simulink model "orion_casestudy_4"  (R2023a)
settings: Solver=VariableStepAuto  StartTime=0.0  StopTime=30  RelTol=1e-3
InitFcn:
  | RandStream.setGlobalStream(RandStream('mt19937ar','seed',sum(100*clock)));
undefined symbols (not defined in the file or in its folder): m, n
(part 1 of 2)
settings Model: Creator=simon  LastModifiedBy=simon
settings OptimizationCC: AccelVerboseBuild=on
settings DebuggingCC: UnderSpecifiedDataTypeMsg=warning  UnderSpecifiedDimensionMsg=warning

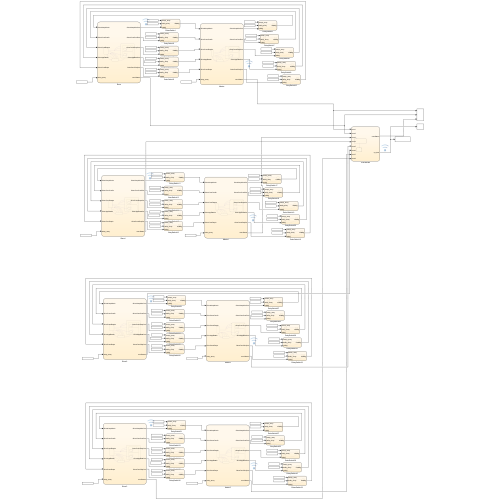
[thumbnail: Simulink's stored preview of the top-level diagram]
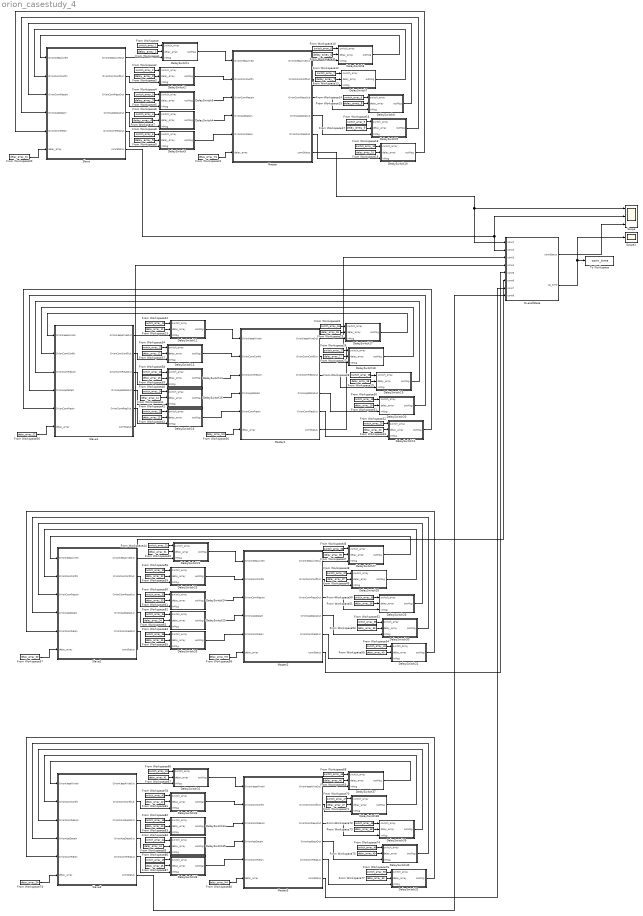
== system orion_casestudy_4 ==
  DelaySwitch1 : Stateflow chart  TreatAsAtomicUnit=on
  DelaySwitch10 : Stateflow chart  TreatAsAtomicUnit=on
  DelaySwitch11 : Stateflow chart  TreatAsAtomicUnit=on
  DelaySwitch12 : Stateflow chart  TreatAsAtomicUnit=on
  DelaySwitch13 : Stateflow chart  TreatAsAtomicUnit=on
  DelaySwitch14 : Stateflow chart  TreatAsAtomicUnit=on
  DelaySwitch15 : Stateflow chart  TreatAsAtomicUnit=on
  DelaySwitch16 : Stateflow chart  TreatAsAtomicUnit=on
  DelaySwitch17 : Stateflow chart  TreatAsAtomicUnit=on
  DelaySwitch18 : Stateflow chart  TreatAsAtomicUnit=on
  DelaySwitch19 : Stateflow chart  TreatAsAtomicUnit=on
  DelaySwitch2 : Stateflow chart  TreatAsAtomicUnit=on
  DelaySwitch20 : Stateflow chart  TreatAsAtomicUnit=on
  DelaySwitch21 : Stateflow chart  TreatAsAtomicUnit=on
  DelaySwitch22 : Stateflow chart  TreatAsAtomicUnit=on
  DelaySwitch23 : Stateflow chart  TreatAsAtomicUnit=on
  DelaySwitch24 : Stateflow chart  TreatAsAtomicUnit=on
  DelaySwitch25 : Stateflow chart  TreatAsAtomicUnit=on
  DelaySwitch26 : Stateflow chart  TreatAsAtomicUnit=on
  DelaySwitch27 : Stateflow chart  TreatAsAtomicUnit=on
  DelaySwitch28 : Stateflow chart  TreatAsAtomicUnit=on
  DelaySwitch29 : Stateflow chart  TreatAsAtomicUnit=on
  DelaySwitch3 : Stateflow chart  TreatAsAtomicUnit=on
  DelaySwitch30 : Stateflow chart  TreatAsAtomicUnit=on
  DelaySwitch31 : Stateflow chart  TreatAsAtomicUnit=on
  DelaySwitch32 : Stateflow chart  TreatAsAtomicUnit=on
  DelaySwitch33 : Stateflow chart  TreatAsAtomicUnit=on
  DelaySwitch34 : Stateflow chart  TreatAsAtomicUnit=on
  DelaySwitch35 : Stateflow chart  TreatAsAtomicUnit=on
  DelaySwitch36 : Stateflow chart  TreatAsAtomicUnit=on
  DelaySwitch37 : Stateflow chart  TreatAsAtomicUnit=on
  DelaySwitch38 : Stateflow chart  TreatAsAtomicUnit=on
  DelaySwitch39 : Stateflow chart  TreatAsAtomicUnit=on
  DelaySwitch4 : Stateflow chart  TreatAsAtomicUnit=on
  DelaySwitch40 : Stateflow chart  TreatAsAtomicUnit=on
  DelaySwitch5 : Stateflow chart  TreatAsAtomicUnit=on
  DelaySwitch6 : Stateflow chart  TreatAsAtomicUnit=on
  DelaySwitch7 : Stateflow chart  TreatAsAtomicUnit=on
  DelaySwitch8 : Stateflow chart  TreatAsAtomicUnit=on
  DelaySwitch9 : Stateflow chart  TreatAsAtomicUnit=on
  From Workspace : FromWorkspace  VariableName=switch_array_1  SampleTime=-1  Interpolate=off  ZeroCross=off  OutputAfterFinalValue=Holding final value
  From Workspace1 : FromWorkspace  VariableName=delay_array_1  SampleTime=-1  Interpolate=off  ZeroCross=off  OutputAfterFinalValue=Holding final value
  From Workspace10 : FromWorkspace  VariableName=switch_array_6  SampleTime=-1  Interpolate=off  ZeroCross=off  OutputAfterFinalValue=Holding final value
  From Workspace11 : FromWorkspace  VariableName=delay_array_6  SampleTime=-1  Interpolate=off  ZeroCross=off  OutputAfterFinalValue=Holding final value
  From Workspace12 : FromWorkspace  VariableName=switch_array_7  SampleTime=-1  Interpolate=off  ZeroCross=off  OutputAfterFinalValue=Holding final value
  From Workspace13 : FromWorkspace  VariableName=delay_array_7  SampleTime=-1  Interpolate=off  ZeroCross=off  OutputAfterFinalValue=Holding final value
  From Workspace14 : FromWorkspace  VariableName=switch_array_8  SampleTime=-1  Interpolate=off  ZeroCross=off  OutputAfterFinalValue=Holding final value
  From Workspace15 : FromWorkspace  VariableName=delay_array_8  SampleTime=-1  Interpolate=off  ZeroCross=off  OutputAfterFinalValue=Holding final value
  From Workspace16 : FromWorkspace  VariableName=switch_array_9  SampleTime=-1  Interpolate=off  ZeroCross=off  OutputAfterFinalValue=Holding final value
  From Workspace17 : FromWorkspace  VariableName=delay_array_9  SampleTime=-1  Interpolate=off  ZeroCross=off  OutputAfterFinalValue=Holding final value
  From Workspace18 : FromWorkspace  VariableName=switch_array_10  SampleTime=-1  Interpolate=off  ZeroCross=off  OutputAfterFinalValue=Holding final value
  From Workspace19 : FromWorkspace  VariableName=delay_array_10  SampleTime=-1  Interpolate=off  ZeroCross=off  OutputAfterFinalValue=Holding final value
  From Workspace2 : FromWorkspace  VariableName=switch_array_2  SampleTime=-1  Interpolate=off  ZeroCross=off  OutputAfterFinalValue=Holding final value
  From Workspace20 : FromWorkspace  VariableName=delay_array_S1  SampleTime=-1  Interpolate=off  ZeroCross=off  OutputAfterFinalValue=Holding final value
  From Workspace21 : FromWorkspace  VariableName=delay_array_M1  SampleTime=-1  Interpolate=off  ZeroCross=off  OutputAfterFinalValue=Holding final value
  From Workspace22 : FromWorkspace  VariableName=switch_array_11  SampleTime=-1  Interpolate=off  ZeroCross=off  OutputAfterFinalValue=Holding final value
  From Workspace23 : FromWorkspace  VariableName=delay_array_11  SampleTime=-1  Interpolate=off  ZeroCross=off  OutputAfterFinalValue=Holding final value
  From Workspace24 : FromWorkspace  VariableName=switch_array_16  SampleTime=-1  Interpolate=off  ZeroCross=off  OutputAfterFinalValue=Holding final value
  From Workspace25 : FromWorkspace  VariableName=delay_array_16  SampleTime=-1  Interpolate=off  ZeroCross=off  OutputAfterFinalValue=Holding final value
  From Workspace26 : FromWorkspace  VariableName=switch_array_17  SampleTime=-1  Interpolate=off  ZeroCross=off  OutputAfterFinalValue=Holding final value
  From Workspace27 : FromWorkspace  VariableName=delay_array_17  SampleTime=-1  Interpolate=off  ZeroCross=off  OutputAfterFinalValue=Holding final value
  From Workspace28 : FromWorkspace  VariableName=switch_array_18  SampleTime=-1  Interpolate=off  ZeroCross=off  OutputAfterFinalValue=Holding final value
  From Workspace29 : FromWorkspace  VariableName=delay_array_18  SampleTime=-1  Interpolate=off  ZeroCross=off  OutputAfterFinalValue=Holding final value
  From Workspace3 : FromWorkspace  VariableName=delay_array_2  SampleTime=-1  Interpolate=off  ZeroCross=off  OutputAfterFinalValue=Holding final value
  From Workspace30 : FromWorkspace  VariableName=switch_array_19  SampleTime=-1  Interpolate=off  ZeroCross=off  OutputAfterFinalValue=Holding final value
  From Workspace31 : FromWorkspace  VariableName=delay_array_19  SampleTime=-1  Interpolate=off  ZeroCross=off  OutputAfterFinalValue=Holding final value
  From Workspace32 : FromWorkspace  VariableName=switch_array_20  SampleTime=-1  Interpolate=off  ZeroCross=off  OutputAfterFinalValue=Holding final value
  From Workspace33 : FromWorkspace  VariableName=delay_array_20  SampleTime=-1  Interpolate=off  ZeroCross=off  OutputAfterFinalValue=Holding final value
  From Workspace34 : FromWorkspace  VariableName=switch_array_12  SampleTime=-1  Interpolate=off  ZeroCross=off  OutputAfterFinalValue=Holding final value
  From Workspace35 : FromWorkspace  VariableName=delay_array_S2  SampleTime=-1  Interpolate=off  ZeroCross=off  OutputAfterFinalValue=Holding final value
  From Workspace36 : FromWorkspace  VariableName=delay_array_M2  SampleTime=-1  Interpolate=off  ZeroCross=off  OutputAfterFinalValue=Holding final value
  From Workspace37 : FromWorkspace  VariableName=delay_array_12  SampleTime=-1  Interpolate=off  ZeroCross=off  OutputAfterFinalValue=Holding final value
  From Workspace38 : FromWorkspace  VariableName=switch_array_13  SampleTime=-1  Interpolate=off  ZeroCross=off  OutputAfterFinalValue=Holding final value
  From Workspace39 : FromWorkspace  VariableName=delay_array_13  SampleTime=-1  Interpolate=off  ZeroCross=off  OutputAfterFinalValue=Holding final value
  From Workspace4 : FromWorkspace  VariableName=switch_array_3  SampleTime=-1  Interpolate=off  ZeroCross=off  OutputAfterFinalValue=Holding final value
  From Workspace40 : FromWorkspace  VariableName=switch_array_14  SampleTime=-1  Interpolate=off  ZeroCross=off  OutputAfterFinalValue=Holding final value
  From Workspace41 : FromWorkspace  VariableName=delay_array_14  SampleTime=-1  Interpolate=off  ZeroCross=off  OutputAfterFinalValue=Holding final value
  From Workspace42 : FromWorkspace  VariableName=switch_array_15  SampleTime=-1  Interpolate=off  ZeroCross=off  OutputAfterFinalValue=Holding final value
  From Workspace43 : FromWorkspace  VariableName=delay_array_15  SampleTime=-1  Interpolate=off  ZeroCross=off  OutputAfterFinalValue=Holding final value
  From Workspace44 : FromWorkspace  VariableName=switch_array_31  SampleTime=-1  Interpolate=off  ZeroCross=off  OutputAfterFinalValue=Holding final value
  From Workspace45 : FromWorkspace  VariableName=delay_array_31  SampleTime=-1  Interpolate=off  ZeroCross=off  OutputAfterFinalValue=Holding final value
  From Workspace46 : FromWorkspace  VariableName=switch_array_36  SampleTime=-1  Interpolate=off  ZeroCross=off  OutputAfterFinalValue=Holding final value
  From Workspace47 : FromWorkspace  VariableName=delay_array_36  SampleTime=-1  Interpolate=off  ZeroCross=off  OutputAfterFinalValue=Holding final value
  From Workspace48 : FromWorkspace  VariableName=switch_array_37  SampleTime=-1  Interpolate=off  ZeroCross=off  OutputAfterFinalValue=Holding final value
  From Workspace49 : FromWorkspace  VariableName=delay_array_37  SampleTime=-1  Interpolate=off  ZeroCross=off  OutputAfterFinalValue=Holding final value
  From Workspace5 : FromWorkspace  VariableName=delay_array_3  SampleTime=-1  Interpolate=off  ZeroCross=off  OutputAfterFinalValue=Holding final value
  From Workspace50 : FromWorkspace  VariableName=switch_array_38  SampleTime=-1  Interpolate=off  ZeroCross=off  OutputAfterFinalValue=Holding final value
  From Workspace51 : FromWorkspace  VariableName=delay_array_38  SampleTime=-1  Interpolate=off  ZeroCross=off  OutputAfterFinalValue=Holding final value
  From Workspace52 : FromWorkspace  VariableName=switch_array_39  SampleTime=-1  Interpolate=off  ZeroCross=off  OutputAfterFinalValue=Holding final value
  From Workspace53 : FromWorkspace  VariableName=delay_array_39  SampleTime=-1  Interpolate=off  ZeroCross=off  OutputAfterFinalValue=Holding final value
  From Workspace54 : FromWorkspace  VariableName=switch_array_40  SampleTime=-1  Interpolate=off  ZeroCross=off  OutputAfterFinalValue=Holding final value
  From Workspace55 : FromWorkspace  VariableName=delay_array_40  SampleTime=-1  Interpolate=off  ZeroCross=off  OutputAfterFinalValue=Holding final value
  From Workspace56 : FromWorkspace  VariableName=switch_array_32  SampleTime=-1  Interpolate=off  ZeroCross=off  OutputAfterFinalValue=Holding final value
  From Workspace57 : FromWorkspace  VariableName=delay_array_S3  SampleTime=-1  Interpolate=off  ZeroCross=off  OutputAfterFinalValue=Holding final value
  From Workspace58 : FromWorkspace  VariableName=delay_array_M3  SampleTime=-1  Interpolate=off  ZeroCross=off  OutputAfterFinalValue=Holding final value
  From Workspace59 : FromWorkspace  VariableName=delay_array_32  SampleTime=-1  Interpolate=off  ZeroCross=off  OutputAfterFinalValue=Holding final value
  From Workspace6 : FromWorkspace  VariableName=switch_array_4  SampleTime=-1  Interpolate=off  ZeroCross=off  OutputAfterFinalValue=Holding final value
  From Workspace60 : FromWorkspace  VariableName=switch_array_33  SampleTime=-1  Interpolate=off  ZeroCross=off  OutputAfterFinalValue=Holding final value
  From Workspace61 : FromWorkspace  VariableName=delay_array_33  SampleTime=-1  Interpolate=off  ZeroCross=off  OutputAfterFinalValue=Holding final value
  From Workspace62 : FromWorkspace  VariableName=switch_array_34  SampleTime=-1  Interpolate=off  ZeroCross=off  OutputAfterFinalValue=Holding final value
  From Workspace63 : FromWorkspace  VariableName=delay_array_34  SampleTime=-1  Interpolate=off  ZeroCross=off  OutputAfterFinalValue=Holding final value
  From Workspace64 : FromWorkspace  VariableName=switch_array_35  SampleTime=-1  Interpolate=off  ZeroCross=off  OutputAfterFinalValue=Holding final value
  From Workspace65 : FromWorkspace  VariableName=delay_array_35  SampleTime=-1  Interpolate=off  ZeroCross=off  OutputAfterFinalValue=Holding final value
  From Workspace66 : FromWorkspace  VariableName=switch_array_41  SampleTime=-1  Interpolate=off  ZeroCross=off  OutputAfterFinalValue=Holding final value
  From Workspace67 : FromWorkspace  VariableName=delay_array_41  SampleTime=-1  Interpolate=off  ZeroCross=off  OutputAfterFinalValue=Holding final value
  From Workspace68 : FromWorkspace  VariableName=switch_array_46  SampleTime=-1  Interpolate=off  ZeroCross=off  OutputAfterFinalValue=Holding final value
  From Workspace69 : FromWorkspace  VariableName=delay_array_46  SampleTime=-1  Interpolate=off  ZeroCross=off  OutputAfterFinalValue=Holding final value
  From Workspace7 : FromWorkspace  VariableName=delay_array_4  SampleTime=-1  Interpolate=off  ZeroCross=off  OutputAfterFinalValue=Holding final value
  From Workspace70 : FromWorkspace  VariableName=switch_array_47  SampleTime=-1  Interpolate=off  ZeroCross=off  OutputAfterFinalValue=Holding final value
  From Workspace71 : FromWorkspace  VariableName=delay_array_47  SampleTime=-1  Interpolate=off  ZeroCross=off  OutputAfterFinalValue=Holding final value
  From Workspace72 : FromWorkspace  VariableName=switch_array_48  SampleTime=-1  Interpolate=off  ZeroCross=off  OutputAfterFinalValue=Holding final value
  From Workspace73 : FromWorkspace  VariableName=delay_array_48  SampleTime=-1  Interpolate=off  ZeroCross=off  OutputAfterFinalValue=Holding final value
  From Workspace74 : FromWorkspace  VariableName=switch_array_49  SampleTime=-1  Interpolate=off  ZeroCross=off  OutputAfterFinalValue=Holding final value
  From Workspace75 : FromWorkspace  VariableName=delay_array_49  SampleTime=-1  Interpolate=off  ZeroCross=off  OutputAfterFinalValue=Holding final value
  From Workspace76 : FromWorkspace  VariableName=switch_array_50  SampleTime=-1  Interpolate=off  ZeroCross=off  OutputAfterFinalValue=Holding final value
  From Workspace77 : FromWorkspace  VariableName=delay_array_50  SampleTime=-1  Interpolate=off  ZeroCross=off  OutputAfterFinalValue=Holding final value
  From Workspace78 : FromWorkspace  VariableName=switch_array_42  SampleTime=-1  Interpolate=off  ZeroCross=off  OutputAfterFinalValue=Holding final value
  From Workspace79 : FromWorkspace  VariableName=delay_array_S4  SampleTime=-1  Interpolate=off  ZeroCross=off  OutputAfterFinalValue=Holding final value
  From Workspace8 : FromWorkspace  VariableName=switch_array_5  SampleTime=-1  Interpolate=off  ZeroCross=off  OutputAfterFinalValue=Holding final value
  From Workspace80 : FromWorkspace  VariableName=delay_array_M4  SampleTime=-1  Interpolate=off  ZeroCross=off  OutputAfterFinalValue=Holding final value
  From Workspace81 : FromWorkspace  VariableName=delay_array_42  SampleTime=-1  Interpolate=off  ZeroCross=off  OutputAfterFinalValue=Holding final value
  From Workspace82 : FromWorkspace  VariableName=switch_array_43  SampleTime=-1  Interpolate=off  ZeroCross=off  OutputAfterFinalValue=Holding final value
  From Workspace83 : FromWorkspace  VariableName=delay_array_43  SampleTime=-1  Interpolate=off  ZeroCross=off  OutputAfterFinalValue=Holding final value
  From Workspace84 : FromWorkspace  VariableName=switch_array_44  SampleTime=-1  Interpolate=off  ZeroCross=off  OutputAfterFinalValue=Holding final value
  From Workspace85 : FromWorkspace  VariableName=delay_array_44  SampleTime=-1  Interpolate=off  ZeroCross=off  OutputAfterFinalValue=Holding final value
  From Workspace86 : FromWorkspace  VariableName=switch_array_45  SampleTime=-1  Interpolate=off  ZeroCross=off  OutputAfterFinalValue=Holding final value
  From Workspace87 : FromWorkspace  VariableName=delay_array_45  SampleTime=-1  Interpolate=off  ZeroCross=off  OutputAfterFinalValue=Holding final value
  From Workspace9 : FromWorkspace  VariableName=delay_array_5  SampleTime=-1  Interpolate=off  ZeroCross=off  OutputAfterFinalValue=Holding final value
  Master : Stateflow chart  TreatAsAtomicUnit=on
      settings: PortSchema="{\"entries\":[{\"content\":{\"sides\":[{\"content\":{\"connectorIds\":[\"In2\",\"In3\",\"In5\",\"In4\",\"In6\",\"In1\"]},\"type\":\"ConnectorPlacement.EquallySpacedRectSide\",\"uuid\":\"93190a42-59cb-4d31-aa72-080cef5549db\"},{\"content\":{\"connectorIds\":[\"Out1\",\"Out2\",\"Out3\",\"Out4\",\"Out5\",\"Out6\"],\"side\":\"RIGHT\"},\"type\":\"ConnectorPlacement.EquallySpacedRectSide\",\"uuid\":\"4a04e977-42e8-4d3e-8e66-86884aeb71d4\"},{\"content\":{\"side\":\"TOP\"},\"type\":\"ConnectorPlacement.EquallySpacedRectSide\",\"uuid\":\"cb7bc3bf-3799-42a3-9f12-c8b4e7be85f7\"},{\"content\":{\"side\":\"BOTTOM\"},\"type\":\"ConnectorPlacement.EquallySpacedRectSide\",\"uuid\":\"934a78a5-af7b-46d0-ad43-c65a76addb63\"}]},\"type\":\"ConnectorPlacement.EquallySpacedConnector\",\"uuid\":\"bab253c4-7746-42e8-9b4d-6fa7ff1cc3b1\"}],\"packageUris\":[\"http://schema.mathworks.com/mf0/Connector/R2020b\"],\"version\":\"1.0\"}"
  Master1 : Stateflow chart  TreatAsAtomicUnit=on
      settings: PortSchema="{\"entries\":[{\"content\":{\"sides\":[{\"content\":{\"connectorIds\":[\"In2\",\"In3\",\"In5\",\"In4\",\"In6\",\"In1\"]},\"type\":\"ConnectorPlacement.EquallySpacedRectSide\",\"uuid\":\"93190a42-59cb-4d31-aa72-080cef5549db\"},{\"content\":{\"connectorIds\":[\"Out1\",\"Out2\",\"Out3\",\"Out4\",\"Out5\",\"Out6\"],\"side\":\"RIGHT\"},\"type\":\"ConnectorPlacement.EquallySpacedRectSide\",\"uuid\":\"4a04e977-42e8-4d3e-8e66-86884aeb71d4\"},{\"content\":{\"side\":\"TOP\"},\"type\":\"ConnectorPlacement.EquallySpacedRectSide\",\"uuid\":\"cb7bc3bf-3799-42a3-9f12-c8b4e7be85f7\"},{\"content\":{\"side\":\"BOTTOM\"},\"type\":\"ConnectorPlacement.EquallySpacedRectSide\",\"uuid\":\"934a78a5-af7b-46d0-ad43-c65a76addb63\"}]},\"type\":\"ConnectorPlacement.EquallySpacedConnector\",\"uuid\":\"bab253c4-7746-42e8-9b4d-6fa7ff1cc3b1\"}],\"packageUris\":[\"http://schema.mathworks.com/mf0/Connector/R2020b\"],\"version\":\"1.0\"}"
  Master2 : Stateflow chart  TreatAsAtomicUnit=on
      settings: PortSchema="{\"entries\":[{\"content\":{\"sides\":[{\"content\":{\"connectorIds\":[\"In2\",\"In3\",\"In5\",\"In4\",\"In6\",\"In1\"]},\"type\":\"ConnectorPlacement.EquallySpacedRectSide\",\"uuid\":\"93190a42-59cb-4d31-aa72-080cef5549db\"},{\"content\":{\"connectorIds\":[\"Out1\",\"Out2\",\"Out3\",\"Out4\",\"Out5\",\"Out6\"],\"side\":\"RIGHT\"},\"type\":\"ConnectorPlacement.EquallySpacedRectSide\",\"uuid\":\"4a04e977-42e8-4d3e-8e66-86884aeb71d4\"},{\"content\":{\"side\":\"TOP\"},\"type\":\"ConnectorPlacement.EquallySpacedRectSide\",\"uuid\":\"cb7bc3bf-3799-42a3-9f12-c8b4e7be85f7\"},{\"content\":{\"side\":\"BOTTOM\"},\"type\":\"ConnectorPlacement.EquallySpacedRectSide\",\"uuid\":\"934a78a5-af7b-46d0-ad43-c65a76addb63\"}]},\"type\":\"ConnectorPlacement.EquallySpacedConnector\",\"uuid\":\"bab253c4-7746-42e8-9b4d-6fa7ff1cc3b1\"}],\"packageUris\":[\"http://schema.mathworks.com/mf0/Connector/R2020b\"],\"version\":\"1.0\"}"
  Master3 : Stateflow chart  TreatAsAtomicUnit=on
      settings: PortSchema="{\"entries\":[{\"content\":{\"sides\":[{\"content\":{\"connectorIds\":[\"In2\",\"In3\",\"In5\",\"In4\",\"In6\",\"In1\"]},\"type\":\"ConnectorPlacement.EquallySpacedRectSide\",\"uuid\":\"93190a42-59cb-4d31-aa72-080cef5549db\"},{\"content\":{\"connectorIds\":[\"Out1\",\"Out2\",\"Out3\",\"Out4\",\"Out5\",\"Out6\"],\"side\":\"RIGHT\"},\"type\":\"ConnectorPlacement.EquallySpacedRectSide\",\"uuid\":\"4a04e977-42e8-4d3e-8e66-86884aeb71d4\"},{\"content\":{\"side\":\"TOP\"},\"type\":\"ConnectorPlacement.EquallySpacedRectSide\",\"uuid\":\"cb7bc3bf-3799-42a3-9f12-c8b4e7be85f7\"},{\"content\":{\"side\":\"BOTTOM\"},\"type\":\"ConnectorPlacement.EquallySpacedRectSide\",\"uuid\":\"934a78a5-af7b-46d0-ad43-c65a76addb63\"}]},\"type\":\"ConnectorPlacement.EquallySpacedConnector\",\"uuid\":\"bab253c4-7746-42e8-9b4d-6fa7ff1cc3b1\"}],\"packageUris\":[\"http://schema.mathworks.com/mf0/Connector/R2020b\"],\"version\":\"1.0\"}"
  OverallState : Stateflow chart  TreatAsAtomicUnit=on
  Scope : Scope  NumInputPorts=3
  Scope1 : Scope
  Slave : Stateflow chart  TreatAsAtomicUnit=on
      settings: PortSchema="{\"entries\":[{\"content\":{\"sides\":[{\"content\":{\"connectorIds\":[\"In1\",\"In5\",\"In3\",\"In2\",\"In4\",\"In6\"]},\"type\":\"ConnectorPlacement.EquallySpacedRectSide\",\"uuid\":\"93190a42-59cb-4d31-aa72-080cef5549db\"},{\"content\":{\"connectorIds\":[\"Out3\",\"Out1\",\"Out2\",\"Out4\",\"Out5\",\"Out6\"],\"side\":\"RIGHT\"},\"type\":\"ConnectorPlacement.EquallySpacedRectSide\",\"uuid\":\"4a04e977-42e8-4d3e-8e66-86884aeb71d4\"},{\"content\":{\"side\":\"TOP\"},\"type\":\"ConnectorPlacement.EquallySpacedRectSide\",\"uuid\":\"cb7bc3bf-3799-42a3-9f12-c8b4e7be85f7\"}]},\"type\":\"ConnectorPlacement.EquallySpacedConnector\",\"uuid\":\"bab253c4-7746-42e8-9b4d-6fa7ff1cc3b1\"}],\"packageUris\":[\"http://schema.mathworks.com/mf0/Connector/R2020b\"],\"version\":\"1.0\"}"
  Slave1 : Stateflow chart  TreatAsAtomicUnit=on
      settings: PortSchema="{\"entries\":[{\"content\":{\"sides\":[{\"content\":{\"connectorIds\":[\"In1\",\"In5\",\"In3\",\"In2\",\"In4\",\"In6\"]},\"type\":\"ConnectorPlacement.EquallySpacedRectSide\",\"uuid\":\"93190a42-59cb-4d31-aa72-080cef5549db\"},{\"content\":{\"connectorIds\":[\"Out3\",\"Out1\",\"Out2\",\"Out4\",\"Out5\",\"Out6\"],\"side\":\"RIGHT\"},\"type\":\"ConnectorPlacement.EquallySpacedRectSide\",\"uuid\":\"4a04e977-42e8-4d3e-8e66-86884aeb71d4\"},{\"content\":{\"side\":\"TOP\"},\"type\":\"ConnectorPlacement.EquallySpacedRectSide\",\"uuid\":\"cb7bc3bf-3799-42a3-9f12-c8b4e7be85f7\"}]},\"type\":\"ConnectorPlacement.EquallySpacedConnector\",\"uuid\":\"bab253c4-7746-42e8-9b4d-6fa7ff1cc3b1\"}],\"packageUris\":[\"http://schema.mathworks.com/mf0/Connector/R2020b\"],\"version\":\"1.0\"}"
  Slave2 : Stateflow chart  TreatAsAtomicUnit=on
      settings: PortSchema="{\"entries\":[{\"content\":{\"sides\":[{\"content\":{\"connectorIds\":[\"In1\",\"In5\",\"In3\",\"In2\",\"In4\",\"In6\"]},\"type\":\"ConnectorPlacement.EquallySpacedRectSide\",\"uuid\":\"93190a42-59cb-4d31-aa72-080cef5549db\"},{\"content\":{\"connectorIds\":[\"Out3\",\"Out1\",\"Out2\",\"Out4\",\"Out5\",\"Out6\"],\"side\":\"RIGHT\"},\"type\":\"ConnectorPlacement.EquallySpacedRectSide\",\"uuid\":\"4a04e977-42e8-4d3e-8e66-86884aeb71d4\"},{\"content\":{\"side\":\"TOP\"},\"type\":\"ConnectorPlacement.EquallySpacedRectSide\",\"uuid\":\"cb7bc3bf-3799-42a3-9f12-c8b4e7be85f7\"}]},\"type\":\"ConnectorPlacement.EquallySpacedConnector\",\"uuid\":\"bab253c4-7746-42e8-9b4d-6fa7ff1cc3b1\"}],\"packageUris\":[\"http://schema.mathworks.com/mf0/Connector/R2020b\"],\"version\":\"1.0\"}"
  Slave3 : Stateflow chart  TreatAsAtomicUnit=on
      settings: PortSchema="{\"entries\":[{\"content\":{\"sides\":[{\"content\":{\"connectorIds\":[\"In1\",\"In5\",\"In3\",\"In2\",\"In4\",\"In6\"]},\"type\":\"ConnectorPlacement.EquallySpacedRectSide\",\"uuid\":\"93190a42-59cb-4d31-aa72-080cef5549db\"},{\"content\":{\"connectorIds\":[\"Out3\",\"Out1\",\"Out2\",\"Out4\",\"Out5\",\"Out6\"],\"side\":\"RIGHT\"},\"type\":\"ConnectorPlacement.EquallySpacedRectSide\",\"uuid\":\"4a04e977-42e8-4d3e-8e66-86884aeb71d4\"},{\"content\":{\"side\":\"TOP\"},\"type\":\"ConnectorPlacement.EquallySpacedRectSide\",\"uuid\":\"cb7bc3bf-3799-42a3-9f12-c8b4e7be85f7\"}]},\"type\":\"ConnectorPlacement.EquallySpacedConnector\",\"uuid\":\"bab253c4-7746-42e8-9b4d-6fa7ff1cc3b1\"}],\"packageUris\":[\"http://schema.mathworks.com/mf0/Connector/R2020b\"],\"version\":\"1.0\"}"
  To Workspace : ToWorkspace  VariableName=conn_time  SaveFormat=Timeseries  SampleTime=-1
  wires:
  Slave/4(OrionAppDataOut) -> DelaySwitch4/3(inMsg)
  Slave/2(OrionConnRespOut) -> DelaySwitch3/3(inMsg)
  Slave/1(OrionConnConfOut) -> DelaySwitch2/3(inMsg)
  Slave/3(OrionKeepAliveOut) -> DelaySwitch1/3(inMsg)
  DelaySwitch3/1(outMsg) -> Master/5(OrionConnRespIn)
  DelaySwitch4/1(outMsg) -> Master/4(OrionAppDataIn)
  DelaySwitch2/1(outMsg) -> Master/3(OrionConnConfIn)
  DelaySwitch1/1(outMsg) -> Master/2(OrionKeepAliveIn)
  DelaySwitch10/1(outMsg) -> Slave/4(OrionConnReqIn)
  DelaySwitch9/1(outMsg) -> Slave/2(OrionAppDataIn)
  DelaySwitch8/1(outMsg) -> Slave/3(OrionConnRespIn)
  DelaySwitch7/1(outMsg) -> Slave/5(OrionConnConfIn)
  DelaySwitch6/1(outMsg) -> Slave/1(OrionKeepAliveIn)
  Master/6(connStatus) -> OverallState/1(conn1), Scope/1
  Slave/6(connStatus) -> Scope/2, OverallState/2(conn2)
  OverallState/1(connStatus) -> Scope/3
  OverallState/2(op_time) -> Scope1/1, To Workspace/1
  From Workspace/1 -> DelaySwitch1/1(switch_array)
  From Workspace1/1 -> DelaySwitch1/2(delay_array)
  From Workspace3/1 -> DelaySwitch2/2(delay_array)
  From Workspace2/1 -> DelaySwitch2/1(switch_array)
  From Workspace4/1 -> DelaySwitch3/1(switch_array)
  From Workspace5/1 -> DelaySwitch3/2(delay_array)
  From Workspace7/1 -> DelaySwitch4/2(delay_array)
  From Workspace6/1 -> DelaySwitch4/1(switch_array)
  From Workspace8/1 -> DelaySwitch5/1(switch_array)
  From Workspace9/1 -> DelaySwitch5/2(delay_array)
  Slave/5(OrionConnReqOut) -> DelaySwitch5/3(inMsg)
  DelaySwitch5/1(outMsg) -> Master/6(OrionConnReqIn)
  From Workspace11/1 -> DelaySwitch6/2(delay_array)
  From Workspace10/1 -> DelaySwitch6/1(switch_array)
  Master/1(OrionKeepAliveOut) -> DelaySwitch6/3(inMsg)
  From Workspace12/1 -> DelaySwitch7/1(switch_array)
  From Workspace13/1 -> DelaySwitch7/2(delay_array)
  From Workspace15/1 -> DelaySwitch8/2(delay_array)
  From Workspace14/1 -> DelaySwitch8/1(switch_array)
  Master/2(OrionConnConfOut) -> DelaySwitch7/3(inMsg)
  Master/3(OrionConnRespOut) -> DelaySwitch8/3(inMsg)
  From Workspace16/1 -> DelaySwitch9/1(switch_array)
  From Workspace17/1 -> DelaySwitch9/2(delay_array)
  From Workspace19/1 -> DelaySwitch10/2(delay_array)
  From Workspace18/1 -> DelaySwitch10/1(switch_array)
  Master/4(OrionAppDataOut) -> DelaySwitch9/3(inMsg)
  Master/5(OrionConnReqOut) -> DelaySwitch10/3(inMsg)
  From Workspace20/1 -> Slave/6(delay_array)
  From Workspace21/1 -> Master/1(delay_array)
  From Workspace36/1 -> Master1/1(delay_array)
  From Workspace35/1 -> Slave1/6(delay_array)
  Master1/5(OrionConnReqOut) -> DelaySwitch12/3(inMsg)
  Master1/4(OrionAppDataOut) -> DelaySwitch20/3(inMsg)
  From Workspace32/1 -> DelaySwitch12/1(switch_array)
  From Workspace33/1 -> DelaySwitch12/2(delay_array)
  From Workspace31/1 -> DelaySwitch20/2(delay_array)
  From Workspace30/1 -> DelaySwitch20/1(switch_array)
  Master1/3(OrionConnRespOut) -> DelaySwitch19/3(inMsg)
  Master1/2(OrionConnConfOut) -> DelaySwitch18/3(inMsg)
  From Workspace28/1 -> DelaySwitch19/1(switch_array)
  From Workspace29/1 -> DelaySwitch19/2(delay_array)
  From Workspace27/1 -> DelaySwitch18/2(delay_array)
  From Workspace26/1 -> DelaySwitch18/1(switch_array)
  Master1/1(OrionKeepAliveOut) -> DelaySwitch17/3(inMsg)
  From Workspace24/1 -> DelaySwitch17/1(switch_array)
  From Workspace25/1 -> DelaySwitch17/2(delay_array)
  DelaySwitch16/1(outMsg) -> Master1/6(OrionConnReqIn)
  Slave1/5(OrionConnReqOut) -> DelaySwitch16/3(inMsg)
  From Workspace43/1 -> DelaySwitch16/2(delay_array)
  From Workspace42/1 -> DelaySwitch16/1(switch_array)
  From Workspace40/1 -> DelaySwitch15/1(switch_array)
  From Workspace41/1 -> DelaySwitch15/2(delay_array)
  From Workspace39/1 -> DelaySwitch14/2(delay_array)
  From Workspace38/1 -> DelaySwitch14/1(switch_array)
  From Workspace34/1 -> DelaySwitch13/1(switch_array)
  From Workspace37/1 -> DelaySwitch13/2(delay_array)
  From Workspace23/1 -> DelaySwitch11/2(delay_array)
  From Workspace22/1 -> DelaySwitch11/1(switch_array)
  Slave1/6(connStatus) -> OverallState/4(conn4)
  Master1/6(connStatus) -> OverallState/3(conn3)
  DelaySwitch17/1(outMsg) -> Slave1/1(OrionKeepAliveIn)
  DelaySwitch18/1(outMsg) -> Slave1/5(OrionConnConfIn)
  DelaySwitch19/1(outMsg) -> Slave1/3(OrionConnRespIn)
  DelaySwitch20/1(outMsg) -> Slave1/2(OrionAppDataIn)
  DelaySwitch12/1(outMsg) -> Slave1/4(OrionConnReqIn)
  DelaySwitch11/1(outMsg) -> Master1/2(OrionKeepAliveIn)
  DelaySwitch13/1(outMsg) -> Master1/3(OrionConnConfIn)
  DelaySwitch15/1(outMsg) -> Master1/4(OrionAppDataIn)
  DelaySwitch14/1(outMsg) -> Master1/5(OrionConnRespIn)
  Slave1/3(OrionKeepAliveOut) -> DelaySwitch11/3(inMsg)
  Slave1/1(OrionConnConfOut) -> DelaySwitch13/3(inMsg)
  Slave1/2(OrionConnRespOut) -> DelaySwitch14/3(inMsg)
  Slave1/4(OrionAppDataOut) -> DelaySwitch15/3(inMsg)
  Slave2/4(OrionAppDataOut) -> DelaySwitch25/3(inMsg)
  Slave2/2(OrionConnRespOut) -> DelaySwitch24/3(inMsg)
  Slave2/1(OrionConnConfOut) -> DelaySwitch23/3(inMsg)
  Slave2/3(OrionKeepAliveOut) -> DelaySwitch21/3(inMsg)
  DelaySwitch24/1(outMsg) -> Master2/5(OrionConnRespIn)
  DelaySwitch25/1(outMsg) -> Master2/4(OrionAppDataIn)
  DelaySwitch23/1(outMsg) -> Master2/3(OrionConnConfIn)
  DelaySwitch21/1(outMsg) -> Master2/2(OrionKeepAliveIn)
  DelaySwitch22/1(outMsg) -> Slave2/4(OrionConnReqIn)
  DelaySwitch30/1(outMsg) -> Slave2/2(OrionAppDataIn)
  DelaySwitch29/1(outMsg) -> Slave2/3(OrionConnRespIn)
  DelaySwitch28/1(outMsg) -> Slave2/5(OrionConnConfIn)
  DelaySwitch27/1(outMsg) -> Slave2/1(OrionKeepAliveIn)
  Master2/6(connStatus) -> OverallState/5(conn5)
  Slave2/6(connStatus) -> OverallState/6(conn6)
  From Workspace44/1 -> DelaySwitch21/1(switch_array)
  From Workspace45/1 -> DelaySwitch21/2(delay_array)
  From Workspace59/1 -> DelaySwitch23/2(delay_array)
  From Workspace56/1 -> DelaySwitch23/1(switch_array)
  From Workspace60/1 -> DelaySwitch24/1(switch_array)
  From Workspace61/1 -> DelaySwitch24/2(delay_array)
  From Workspace63/1 -> DelaySwitch25/2(delay_array)
  From Workspace62/1 -> DelaySwitch25/1(switch_array)
  From Workspace64/1 -> DelaySwitch26/1(switch_array)
  From Workspace65/1 -> DelaySwitch26/2(delay_array)
  Slave2/5(OrionConnReqOut) -> DelaySwitch26/3(inMsg)
  DelaySwitch26/1(outMsg) -> Master2/6(OrionConnReqIn)
  From Workspace47/1 -> DelaySwitch27/2(delay_array)
  From Workspace46/1 -> DelaySwitch27/1(switch_array)
  Master2/1(OrionKeepAliveOut) -> DelaySwitch27/3(inMsg)
  From Workspace48/1 -> DelaySwitch28/1(switch_array)
  From Workspace49/1 -> DelaySwitch28/2(delay_array)
  From Workspace51/1 -> DelaySwitch29/2(delay_array)
  From Workspace50/1 -> DelaySwitch29/1(switch_array)
  Master2/2(OrionConnConfOut) -> DelaySwitch28/3(inMsg)
  Master2/3(OrionConnRespOut) -> DelaySwitch29/3(inMsg)
  From Workspace52/1 -> DelaySwitch30/1(switch_array)
  From Workspace53/1 -> DelaySwitch30/2(delay_array)
  From Workspace55/1 -> DelaySwitch22/2(delay_array)
  From Workspace54/1 -> DelaySwitch22/1(switch_array)
  Master2/4(OrionAppDataOut) -> DelaySwitch30/3(inMsg)
  Master2/5(OrionConnReqOut) -> DelaySwitch22/3(inMsg)
  From Workspace57/1 -> Slave2/6(delay_array)
  From Workspace58/1 -> Master2/1(delay_array)
  From Workspace80/1 -> Master3/1(delay_array)
  From Workspace79/1 -> Slave3/6(delay_array)
  Master3/5(OrionConnReqOut) -> DelaySwitch32/3(inMsg)
  Master3/4(OrionAppDataOut) -> DelaySwitch40/3(inMsg)
  From Workspace76/1 -> DelaySwitch32/1(switch_array)
  From Workspace77/1 -> DelaySwitch32/2(delay_array)
  From Workspace75/1 -> DelaySwitch40/2(delay_array)
  From Workspace74/1 -> DelaySwitch40/1(switch_array)
  Master3/3(OrionConnRespOut) -> DelaySwitch39/3(inMsg)
  Master3/2(OrionConnConfOut) -> DelaySwitch38/3(inMsg)
  From Workspace72/1 -> DelaySwitch39/1(switch_array)
  From Workspace73/1 -> DelaySwitch39/2(delay_array)
  From Workspace71/1 -> DelaySwitch38/2(delay_array)
  From Workspace70/1 -> DelaySwitch38/1(switch_array)
  Master3/1(OrionKeepAliveOut) -> DelaySwitch37/3(inMsg)
  From Workspace68/1 -> DelaySwitch37/1(switch_array)
  From Workspace69/1 -> DelaySwitch37/2(delay_array)
  DelaySwitch36/1(outMsg) -> Master3/6(OrionConnReqIn)
  Slave3/5(OrionConnReqOut) -> DelaySwitch36/3(inMsg)
  From Workspace87/1 -> DelaySwitch36/2(delay_array)
  From Workspace86/1 -> DelaySwitch36/1(switch_array)
  From Workspace84/1 -> DelaySwitch35/1(switch_array)
  From Workspace85/1 -> DelaySwitch35/2(delay_array)
  From Workspace83/1 -> DelaySwitch34/2(delay_array)
  From Workspace82/1 -> DelaySwitch34/1(switch_array)
  From Workspace78/1 -> DelaySwitch33/1(switch_array)
  From Workspace81/1 -> DelaySwitch33/2(delay_array)
  From Workspace67/1 -> DelaySwitch31/2(delay_array)
  From Workspace66/1 -> DelaySwitch31/1(switch_array)
  Slave3/6(connStatus) -> OverallState/8(conn8)
  Master3/6(connStatus) -> OverallState/7(conn7)
  DelaySwitch37/1(outMsg) -> Slave3/1(OrionKeepAliveIn)
  DelaySwitch38/1(outMsg) -> Slave3/5(OrionConnConfIn)
  DelaySwitch39/1(outMsg) -> Slave3/3(OrionConnRespIn)
  DelaySwitch40/1(outMsg) -> Slave3/2(OrionAppDataIn)
  DelaySwitch32/1(outMsg) -> Slave3/4(OrionConnReqIn)
  DelaySwitch31/1(outMsg) -> Master3/2(OrionKeepAliveIn)
  DelaySwitch33/1(outMsg) -> Master3/3(OrionConnConfIn)
  DelaySwitch35/1(outMsg) -> Master3/4(OrionAppDataIn)
  DelaySwitch34/1(outMsg) -> Master3/5(OrionConnRespIn)
  Slave3/3(OrionKeepAliveOut) -> DelaySwitch31/3(inMsg)
  Slave3/1(OrionConnConfOut) -> DelaySwitch33/3(inMsg)
  Slave3/2(OrionConnRespOut) -> DelaySwitch34/3(inMsg)
  Slave3/4(OrionAppDataOut) -> DelaySwitch35/3(inMsg)

== stateflow chart orion_casestudy_4/DelaySwitch3 ==
  state Operation
  state Sending
  (default) -> Operation : {i=0;}
  (junction 7) -> Operation [order 2]
  Sending -> Operation : after(delay_array(i),msec)
      | {receive(inMsg);outMsg.data=0;send(outMsg);}
  Operation -> (junction 7) : inMsg{i = i + 1;}
  (junction 7) -> Sending [order 1] : [switch_array(i)==0]
  data: switch_array input; delay_array input; outMsg output; inMsg input; i local

== stateflow chart orion_casestudy_4/DelaySwitch4 ==
  state Operation
  state Sending
  (default) -> Operation : {i=0;}
  (junction 7) -> Operation [order 2]
  Sending -> Operation : after(delay_array(i),msec)
      | {receive(inMsg);outMsg.data=0;send(outMsg);}
  Operation -> (junction 7) : inMsg{i = i + 1;}
  (junction 7) -> Sending [order 1] : [switch_array(i)==0]
  data: switch_array input; delay_array input; outMsg output; inMsg input; i local

== stateflow chart orion_casestudy_4/DelaySwitch5 ==
  state Operation
  state Sending
  (default) -> Operation : {i=0;}
  (junction 7) -> Operation [order 2]
  Sending -> Operation : after(delay_array(i),msec)
      | {receive(inMsg);outMsg.data=0;send(outMsg);}
  Operation -> (junction 7) : inMsg{i = i + 1;}
  (junction 7) -> Sending [order 1] : [switch_array(i)==0]
  data: switch_array input; delay_array input; outMsg output; inMsg input; i local

== stateflow chart orion_casestudy_4/DelaySwitch6 ==
  state Operation
  state Sending
  (default) -> Operation : {i=0;}
  (junction 7) -> Operation [order 2]
  Sending -> Operation : after(delay_array(i),msec)
      | {receive(inMsg);outMsg.data=0;send(outMsg);}
  Operation -> (junction 7) : inMsg{i = i + 1;}
  (junction 7) -> Sending [order 1] : [switch_array(i)==0]
  data: switch_array input; delay_array input; outMsg output; inMsg input; i local

== stateflow chart orion_casestudy_4/Slave ==
  settings: updateMethod=CONTINUOUS
  state Connected
    entry:
    connStatus=2;
    state KeepAliveSendTimeout [parallel]
      settings: executionOrder=1
      state KeepAliveSend
      (default) -> KeepAliveSend
      KeepAliveSend -> KeepAliveSend [order 1] : after(delay_array(i)*5,msec)
          |  {OrionKeepAliveOut.data=0;
          | send(OrionKeepAliveOut);i = i + 1;}
      KeepAliveSend -> KeepAliveSend [order 2] : SendDataIn
          | {OrionAppDataOut.data=0;
          | send(OrionAppDataOut);}
    state KeepAliveRecieveTimeout [parallel]
      settings: executionOrder=2
      state KeepAlineRec
      (default) -> KeepAlineRec
      KeepAlineRec -> KeepAlineRec [order 2] : OrionKeepAliveIn
      KeepAlineRec -> KeepAlineRec [order 3] : OrionAppDataIn
  state Closed
    entry:
    connStatus=0;
  state Connecting
    entry:
    connStatus=1;
  Connected -> (junction 6) [order 2] : OrionConnRespIn
  Connected -> (junction 6) [order 3] : OrionConnReqIn
  (default) -> Closed : {i=1;}
  (junction 6) -> Closed
  Connected -> (junction 6) [order 1] : OrionConnConfIn
  KeepAlineRec -> Closed [order 1] : after(delay_array(i)*5,msec)
      | {i = i + 1;}
  Connecting -> (junction 36) [order 6] : OrionAppDataIn
  Connecting -> (junction 36) [order 5] : OrionConnReqIn
  (junction 36) -> Closed
  Connecting -> (junction 36) [order 4] : OrionConnRespIn
  Connecting -> (junction 36) [order 3] : OrionKeepAliveIn
  Closed -> Connecting : OrionConnReqIn
      | {OrionConnRespOut.data=0;
      | send(OrionConnRespOut);}
  Connecting -> Closed [order 1] : after(delay_array(i)*5,msec)
      | {i = i + 1;}
  Connecting -> Connected [order 2] : OrionConnConfIn{OrionConnConfOut.data=0;send(OrionConnConfOut);}
  data: OrionKeepAliveIn input; OrionConnConfOut output; OrionConnRespOut output; OrionKeepAliveOut output; OrionAppDataOut output; OrionAppDataIn input; OrionConnRespIn input; OrionConnReqIn input; OrionConnReqOut output size=1; connStatus output; SendDataIn local; OrionConnConfIn input; delay_array input; i local

== stateflow chart orion_casestudy_4/DelaySwitch7 ==
  state Operation
  state Sending
  (default) -> Operation : {i=0;}
  (junction 7) -> Operation [order 2]
  Sending -> Operation : after(delay_array(i),msec)
      | {receive(inMsg);outMsg.data=0;send(outMsg);}
  Operation -> (junction 7) : inMsg{i = i + 1;}
  (junction 7) -> Sending [order 1] : [switch_array(i)==0]
  data: switch_array input; delay_array input; outMsg output; inMsg input; i local

== stateflow chart orion_casestudy_4/DelaySwitch8 ==
  state Operation
  state Sending
  (default) -> Operation : {i=0;}
  (junction 7) -> Operation [order 2]
  Sending -> Operation : after(delay_array(i),msec)
      | {receive(inMsg);outMsg.data=0;send(outMsg);}
  Operation -> (junction 7) : inMsg{i = i + 1;}
  (junction 7) -> Sending [order 1] : [switch_array(i)==0]
  data: switch_array input; delay_array input; outMsg output; inMsg input; i local

== stateflow chart orion_casestudy_4/DelaySwitch9 ==
  state Operation
  state Sending
  (default) -> Operation : {i=0;}
  (junction 7) -> Operation [order 2]
  Sending -> Operation : after(delay_array(i),msec)
      | {receive(inMsg);outMsg.data=0;send(outMsg);}
  Operation -> (junction 7) : inMsg{i = i + 1;}
  (junction 7) -> Sending [order 1] : [switch_array(i)==0]
  data: switch_array input; delay_array input; outMsg output; inMsg input; i local

== stateflow chart orion_casestudy_4/DelaySwitch10 ==
  state Operation
  state Sending
  (default) -> Operation : {i=0;}
  (junction 7) -> Operation [order 2]
  Sending -> Operation : after(delay_array(i),msec)
      | {receive(inMsg);outMsg.data=0;send(outMsg);}
  Operation -> (junction 7) : inMsg{i = i + 1;}
  (junction 7) -> Sending [order 1] : [switch_array(i)==0]
  data: switch_array input; delay_array input; outMsg output; inMsg input; i local

== stateflow chart orion_casestudy_4/OverallState ==
  settings: updateMethod=CONTINUOUS
  state NotConnected
    op_time=temporalCount(msec);
  state Connected
    entry:
    connStatus=1;
  (default) -> NotConnected : {connStatus=0;
      | op_time=0;}
  NotConnected -> Connected : [(conn1==2 && conn2==2) ||  (conn3==2 && conn4==2) ||  (conn5==2 && conn6==2) ||  (conn7==2 && conn8==2)]
  data: conn1 input; conn2 input; connStatus output; op_time output; conn3 input; conn4 input; conn5 input; conn6 input; conn7 input; conn8 input

== stateflow chart orion_casestudy_4/DelaySwitch11 ==
  state Operation
  state Sending
  (default) -> Operation : {i=0;}
  (junction 7) -> Operation [order 2]
  Sending -> Operation : after(delay_array(i),msec)
      | {receive(inMsg);outMsg.data=0;send(outMsg);}
  Operation -> (junction 7) : inMsg{i = i + 1;}
  (junction 7) -> Sending [order 1] : [switch_array(i)==0]
  data: switch_array input; delay_array input; outMsg output; inMsg input; i local

== stateflow chart orion_casestudy_4/DelaySwitch12 ==
  state Operation
  state Sending
  (default) -> Operation : {i=0;}
  (junction 7) -> Operation [order 2]
  Sending -> Operation : after(delay_array(i),msec)
      | {receive(inMsg);outMsg.data=0;send(outMsg);}
  Operation -> (junction 7) : inMsg{i = i + 1;}
  (junction 7) -> Sending [order 1] : [switch_array(i)==0]
  data: switch_array input; delay_array input; outMsg output; inMsg input; i local

== stateflow chart orion_casestudy_4/DelaySwitch13 ==
  state Operation
  state Sending
  (default) -> Operation : {i=0;}
  (junction 7) -> Operation [order 2]
  Sending -> Operation : after(delay_array(i),msec)
      | {receive(inMsg);outMsg.data=0;send(outMsg);}
  Operation -> (junction 7) : inMsg{i = i + 1;}
  (junction 7) -> Sending [order 1] : [switch_array(i)==0]
  data: switch_array input; delay_array input; outMsg output; inMsg input; i local

== stateflow chart orion_casestudy_4/DelaySwitch14 ==
  state Operation
  state Sending
  (default) -> Operation : {i=0;}
  (junction 7) -> Operation [order 2]
  Sending -> Operation : after(delay_array(i),msec)
      | {receive(inMsg);outMsg.data=0;send(outMsg);}
  Operation -> (junction 7) : inMsg{i = i + 1;}
  (junction 7) -> Sending [order 1] : [switch_array(i)==0]
  data: switch_array input; delay_array input; outMsg output; inMsg input; i local

== stateflow chart orion_casestudy_4/DelaySwitch15 ==
  state Operation
  state Sending
  (default) -> Operation : {i=0;}
  (junction 7) -> Operation [order 2]
  Sending -> Operation : after(delay_array(i),msec)
      | {receive(inMsg);outMsg.data=0;send(outMsg);}
  Operation -> (junction 7) : inMsg{i = i + 1;}
  (junction 7) -> Sending [order 1] : [switch_array(i)==0]
  data: switch_array input; delay_array input; outMsg output; inMsg input; i local

== stateflow chart orion_casestudy_4/DelaySwitch16 ==
  state Operation
  state Sending
  (default) -> Operation : {i=0;}
  (junction 7) -> Operation [order 2]
  Sending -> Operation : after(delay_array(i),msec)
      | {receive(inMsg);outMsg.data=0;send(outMsg);}
  Operation -> (junction 7) : inMsg{i = i + 1;}
  (junction 7) -> Sending [order 1] : [switch_array(i)==0]
  data: switch_array input; delay_array input; outMsg output; inMsg input; i local

== stateflow chart orion_casestudy_4/DelaySwitch17 ==
  state Operation
  state Sending
  (default) -> Operation : {i=0;}
  (junction 7) -> Operation [order 2]
  Sending -> Operation : after(delay_array(i),msec)
      | {receive(inMsg);outMsg.data=0;send(outMsg);}
  Operation -> (junction 7) : inMsg{i = i + 1;}
  (junction 7) -> Sending [order 1] : [switch_array(i)==0]
  data: switch_array input; delay_array input; outMsg output; inMsg input; i local

== stateflow chart orion_casestudy_4/DelaySwitch18 ==
  state Operation
  state Sending
  (default) -> Operation : {i=0;}
  (junction 7) -> Operation [order 2]
  Sending -> Operation : after(delay_array(i),msec)
      | {receive(inMsg);outMsg.data=0;send(outMsg);}
  Operation -> (junction 7) : inMsg{i = i + 1;}
  (junction 7) -> Sending [order 1] : [switch_array(i)==0]
  data: switch_array input; delay_array input; outMsg output; inMsg input; i local

== stateflow chart orion_casestudy_4/DelaySwitch19 ==
  state Operation
  state Sending
  (default) -> Operation : {i=0;}
  (junction 7) -> Operation [order 2]
  Sending -> Operation : after(delay_array(i),msec)
      | {receive(inMsg);outMsg.data=0;send(outMsg);}
  Operation -> (junction 7) : inMsg{i = i + 1;}
  (junction 7) -> Sending [order 1] : [switch_array(i)==0]
  data: switch_array input; delay_array input; outMsg output; inMsg input; i local

== stateflow chart orion_casestudy_4/DelaySwitch20 ==
  state Operation
  state Sending
  (default) -> Operation : {i=0;}
  (junction 7) -> Operation [order 2]
  Sending -> Operation : after(delay_array(i),msec)
      | {receive(inMsg);outMsg.data=0;send(outMsg);}
  Operation -> (junction 7) : inMsg{i = i + 1;}
  (junction 7) -> Sending [order 1] : [switch_array(i)==0]
  data: switch_array input; delay_array input; outMsg output; inMsg input; i local

== stateflow chart orion_casestudy_4/Master1 ==
  settings: updateMethod=CONTINUOUS
  state Connected
    entry:
    connStatus=2;
    state KeepAliveSendTimeout [parallel]
      settings: executionOrder=1
      state KeepAliveSend
      (default) -> KeepAliveSend
      KeepAliveSend -> KeepAliveSend [order 1] : after(delay_array(i)*5,msec)
          | {OrionKeepAliveOut.data=0;
          | send(OrionKeepAliveOut);
          | i = i + 1;}
      KeepAliveSend -> KeepAliveSend [order 2] : SendDataIn
          | {OrionAppDataOut.data=0;
          | send(OrionAppDataOut);}
    state KeepAliveRecieveTimeout [parallel]
      settings: executionOrder=2
      state KeepAlineRec
      (default) -> KeepAlineRec
      KeepAlineRec -> KeepAlineRec [order 2] : OrionKeepAliveIn
      KeepAlineRec -> KeepAlineRec [order 3] : OrionAppDataIn
  state Closed
    entry:
    connStatus=0;
  state Connecting
    entry:
    connStatus=1;
  Connected -> (junction 6) [order 1] : OrionConnConfIn
  (default) -> Closed : {i=1;}
  Connected -> (junction 6) [order 2] : OrionConnRespIn
  Connected -> (junction 6) [order 3] : OrionConnReqIn
  (junction 6) -> Closed
  KeepAlineRec -> Closed [order 1] : after(delay_array(i)*5,msec)
      | {i = i + 1;}
  Connecting -> (junction 36) [order 5] : OrionConnReqIn
  (junction 36) -> Closed
  Connecting -> (junction 36) [order 4] : OrionConnRespIn
  Connecting -> (junction 36) [order 2] : OrionKeepAliveIn
  Connecting -> Closed [order 3] : after(delay_array(i)*5,msec)
      | {i = i + 1;}
  Closed -> Connecting [order 2] : after(delay_array(i)*5,msec)
      | {OrionConnReqOut.data=0;send(OrionConnReqOut);i = i + 1;}
  Closed -> Connecting [order 1] : OrionConnReqIn
      | {OrionConnRespOut.data=0;send(OrionConnRespOut);}
  Connecting -> Connected [order 1] : OrionConnRespIn
      | {OrionConnConfOut.data=0;
      | send(OrionConnConfOut);}
  data: delay_array input; OrionKeepAliveOut output; OrionKeepAliveIn input; OrionConnConfOut output; OrionConnConfIn input; OrionConnRespOut output; OrionAppDataOut output; OrionAppDataIn input; OrionConnRespIn input; OrionConnReqIn input; OrionConnReqOut output; connStatus output; SendDataIn local; i local

== stateflow chart orion_casestudy_4/Slave1 ==
  settings: updateMethod=CONTINUOUS
  state Connected
    entry:
    connStatus=2;
    state KeepAliveSendTimeout [parallel]
      settings: executionOrder=1
      state KeepAliveSend
      (default) -> KeepAliveSend
      KeepAliveSend -> KeepAliveSend [order 1] : after(delay_array(i)*5,msec)
          |  {OrionKeepAliveOut.data=0;
          | send(OrionKeepAliveOut);i = i + 1;}
      KeepAliveSend -> KeepAliveSend [order 2] : SendDataIn
          | {OrionAppDataOut.data=0;
          | send(OrionAppDataOut);}
    state KeepAliveRecieveTimeout [parallel]
      settings: executionOrder=2
      state KeepAlineRec
      (default) -> KeepAlineRec
      KeepAlineRec -> KeepAlineRec [order 2] : OrionKeepAliveIn
      KeepAlineRec -> KeepAlineRec [order 3] : OrionAppDataIn
  state Closed
    entry:
    connStatus=0;
  state Connecting
    entry:
    connStatus=1;
  Connected -> (junction 6) [order 2] : OrionConnRespIn
  Connected -> (junction 6) [order 3] : OrionConnReqIn
  (default) -> Closed : {i=1;}
  (junction 6) -> Closed
  Connected -> (junction 6) [order 1] : OrionConnConfIn
  KeepAlineRec -> Closed [order 1] : after(delay_array(i)*5,msec)
      | {i = i + 1;}
  Connecting -> (junction 36) [order 6] : OrionAppDataIn
  Connecting -> (junction 36) [order 5] : OrionConnReqIn
  (junction 36) -> Closed
  Connecting -> (junction 36) [order 4] : OrionConnRespIn
  Connecting -> (junction 36) [order 3] : OrionKeepAliveIn
  Closed -> Connecting : OrionConnReqIn
      | {OrionConnRespOut.data=0;
      | send(OrionConnRespOut);}
  Connecting -> Closed [order 1] : after(delay_array(i)*5,msec)
      | {i = i + 1;}
  Connecting -> Connected [order 2] : OrionConnConfIn{OrionConnConfOut.data=0;send(OrionConnConfOut);}
  data: OrionKeepAliveIn input; OrionConnConfOut output; OrionConnRespOut output; OrionKeepAliveOut output; OrionAppDataOut output; OrionAppDataIn input; OrionConnRespIn input; OrionConnReqIn input; OrionConnReqOut output size=1; connStatus output; SendDataIn local; OrionConnConfIn input; delay_array input; i local

== stateflow chart orion_casestudy_4/DelaySwitch21 ==
  state Operation
  state Sending
  (default) -> Operation : {i=0;}
  (junction 7) -> Operation [order 2]
  Sending -> Operation : after(delay_array(i),msec)
      | {receive(inMsg);outMsg.data=0;send(outMsg);}
  Operation -> (junction 7) : inMsg{i = i + 1;}
  (junction 7) -> Sending [order 1] : [switch_array(i)==0]
  data: switch_array input; delay_array input; outMsg output; inMsg input; i local

== stateflow chart orion_casestudy_4/DelaySwitch22 ==
  state Operation
  state Sending
  (default) -> Operation : {i=0;}
  (junction 7) -> Operation [order 2]
  Sending -> Operation : after(delay_array(i),msec)
      | {receive(inMsg);outMsg.data=0;send(outMsg);}
  Operation -> (junction 7) : inMsg{i = i + 1;}
  (junction 7) -> Sending [order 1] : [switch_array(i)==0]
  data: switch_array input; delay_array input; outMsg output; inMsg input; i local

== stateflow chart orion_casestudy_4/DelaySwitch23 ==
  state Operation
  state Sending
  (default) -> Operation : {i=0;}
  (junction 7) -> Operation [order 2]
  Sending -> Operation : after(delay_array(i),msec)
      | {receive(inMsg);outMsg.data=0;send(outMsg);}
  Operation -> (junction 7) : inMsg{i = i + 1;}
  (junction 7) -> Sending [order 1] : [switch_array(i)==0]
  data: switch_array input; delay_array input; outMsg output; inMsg input; i local

== stateflow chart orion_casestudy_4/DelaySwitch24 ==
  state Operation
  state Sending
  (default) -> Operation : {i=0;}
  (junction 7) -> Operation [order 2]
  Sending -> Operation : after(delay_array(i),msec)
      | {receive(inMsg);outMsg.data=0;send(outMsg);}
  Operation -> (junction 7) : inMsg{i = i + 1;}
  (junction 7) -> Sending [order 1] : [switch_array(i)==0]
  data: switch_array input; delay_array input; outMsg output; inMsg input; i local
